simulink model "test01"  (R2025b)
settings: Solver=VariableStepAuto  StartTime=0.0  StopTime=60  RelTol=1e-3
settings Model: Creator=sanborkl  LastModifiedBy=sanborkl

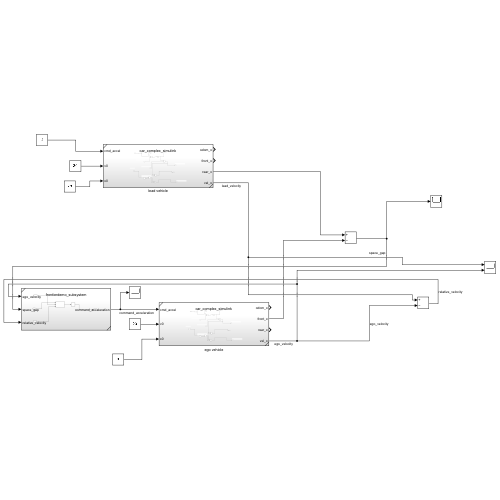
[thumbnail: Simulink's stored preview of the top-level diagram]
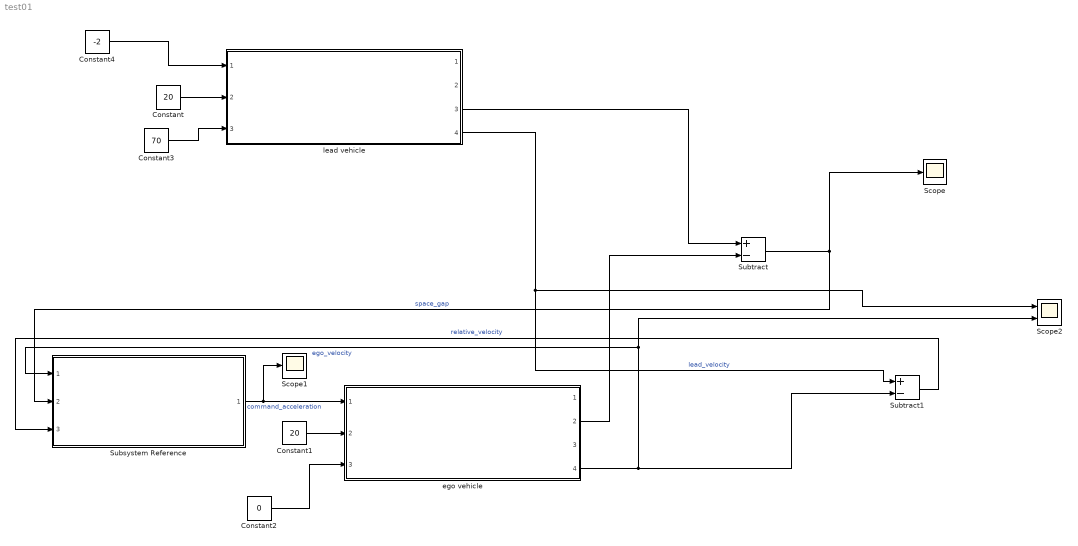
== system test01 ==
  Constant : Constant  Value=20
  Constant1 : Constant  Value=20
  Constant2 : Constant  Value=0
  Constant3 : Constant  Value=70
  Constant4 : Constant  Value=-2
  Scope : Scope
      settings: ActiveDisplayYMinimum=3.0001370188264627  ActiveDisplayYMaximum=72.999984775685945
  Scope1 : Scope
      settings: ActiveDisplayYMinimum=-2.14324906625149  ActiveDisplayYMaximum=0.23813254119485963
  Scope2 : Scope  NumInputPorts=2
      settings: ActiveDisplayYMinimum=-2.4999999999999996  ActiveDisplayYMaximum=22.5  DataLoggingVariableName=ScopeData2
  Subsystem Reference : Subsystem  ReferencedSubsystem=frontierdemo_subsystem
  Subtract : Sum  Inputs=+-
  Subtract1 : Sum  Inputs=+-
  ego vehicle : Subsystem  ReferencedSubsystem=car_complex_simulink
  lead vehicle : Subsystem  ReferencedSubsystem=car_complex_simulink
  wires:
  Subsystem Reference/1 -> Scope1/1, ego vehicle/1  "command_acceleration"
  lead vehicle/3 -> Subtract/1
  ego vehicle/2 -> Subtract/2
  Subtract/1 -> Subsystem Reference/2, Scope/1  "space_gap"
  lead vehicle/4 -> Scope2/1, Subtract1/1  "lead_velocity"
  ego vehicle/4 -> Scope2/2, Subsystem Reference/1, Subtract1/2  "ego_velocity"
  Subtract1/1 -> Subsystem Reference/3  "relative_velocity"
  Constant/1 -> lead vehicle/2
  Constant1/1 -> ego vehicle/2
  Constant2/1 -> ego vehicle/3
  Constant3/1 -> lead vehicle/3
  Constant4/1 -> lead vehicle/1
